simulink model "ob_1_model"  (R2018b)
settings: Solver=VariableStepAuto  StartTime=0.0  StopTime=10.0  RelTol=1e-3
values from neighbouring files (symbols this model uses):
  K = 2    [ob_1.m]    (also in ob_2.m; ob_3.m)
  T_1 = 1    [ob_1.m]    (also in ob_2.m; ob_3.m)
  T_1_a = 0    [ob_1.m]    (also in ob_2.m; ob_3.m)
  T_1_b = T_1/10    (= 0.1)    [ob_1.m]    (also in ob_2.m; ob_3.m)
  T_1_c = T_1/2    (= 0.5)    [ob_1.m]    (also in ob_2.m; ob_3.m)
  T_1_d = T_1*1.05    (= 1.05)    [ob_1.m]    (also in ob_2.m; ob_3.m)
  T_2_a = 0    [ob_1.m]    (also in ob_2.m)
  T_2_b = T_i/100    (= 0.01)    [ob_1.m]    (also in ob_2.m)
  T_2_c = T_i/10    (= 0.1)    [ob_1.m]    (also in ob_2.m)
  T_2_d = T_i*0.99    (= 0.99)    [ob_1.m]    (also in ob_2.m)
  T_2_e = 10*T_i    (= 10)    [ob_1.m]    (also in ob_2.m)
  T_3_a = 0.0001    [ob_1.m]    (also in ob_2.m)
  T_3_b = T_d/100    (= 0.01)    [ob_1.m]    (also in ob_2.m)
  T_3_c = T_d/10    (= 0.1)    [ob_1.m]    (also in ob_2.m)
  T_3_d = T_d*0.99    (= 0.99)    [ob_1.m]    (also in ob_2.m)
  T_d = 1    [ob_1.m]    (also in ob_2.m; ob_3.m = 2.5)
  T_i = 1    [ob_1.m]    (also in ob_2.m)
settings Model: Creator=root  LastModifiedBy=root

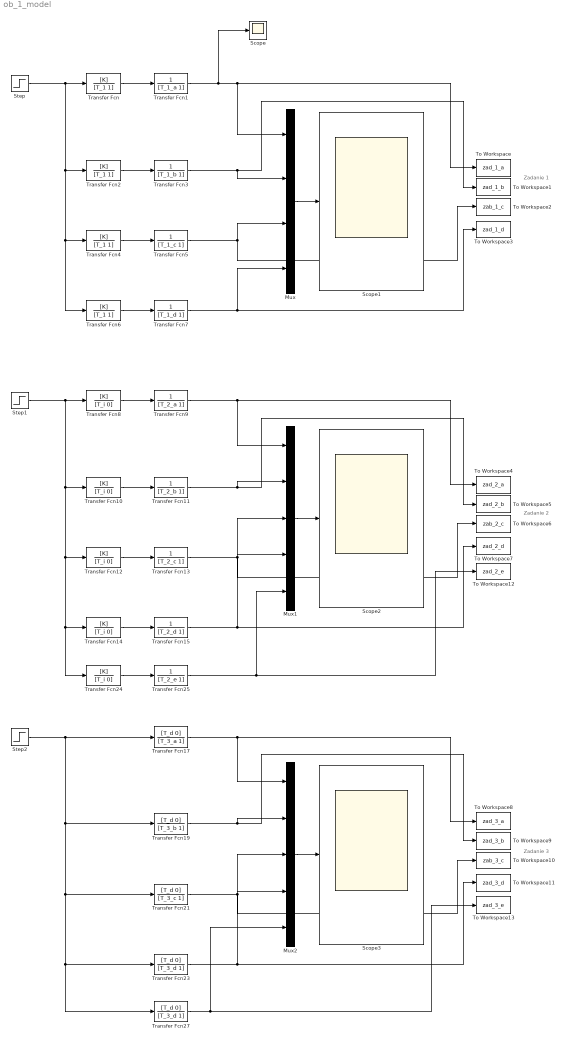
== system ob_1_model ==
  note: Zadanie 3
  note: Zadanie 2
  note: Zadanie 1
  Mux : Mux
  Mux1 : Mux  Inputs=5
  Mux2 : Mux  Inputs=5
  Scope{,1..3} (4 alike) : Scope
  Step : Step  SampleTime=0
  Step1 : Step  SampleTime=0
  Step2 : Step  SampleTime=0
  To Workspace : ToWorkspace  VariableName=zad_1_a  SaveFormat=Timeseries  SampleTime=-1
  To Workspace1 : ToWorkspace  VariableName=zad_1_b  SaveFormat=Timeseries  SampleTime=-1
  To Workspace10 : ToWorkspace  VariableName=zab_3_c  SaveFormat=Timeseries  SampleTime=-1
  To Workspace11 : ToWorkspace  VariableName=zad_3_d  SaveFormat=Timeseries  SampleTime=-1
  To Workspace12 : ToWorkspace  VariableName=zad_2_e  SaveFormat=Timeseries  SampleTime=-1
  To Workspace13 : ToWorkspace  VariableName=zad_3_e  SaveFormat=Timeseries  SampleTime=-1
  To Workspace2 : ToWorkspace  VariableName=zab_1_c  SaveFormat=Timeseries  SampleTime=-1
  To Workspace3 : ToWorkspace  VariableName=zad_1_d  SaveFormat=Timeseries  SampleTime=-1
  To Workspace4 : ToWorkspace  VariableName=zad_2_a  SaveFormat=Timeseries  SampleTime=-1
  To Workspace5 : ToWorkspace  VariableName=zad_2_b  SaveFormat=Timeseries  SampleTime=-1
  To Workspace6 : ToWorkspace  VariableName=zab_2_c  SaveFormat=Timeseries  SampleTime=-1
  To Workspace7 : ToWorkspace  VariableName=zad_2_d  SaveFormat=Timeseries  SampleTime=-1
  To Workspace8 : ToWorkspace  VariableName=zad_3_a  SaveFormat=Timeseries  SampleTime=-1
  To Workspace9 : ToWorkspace  VariableName=zad_3_b  SaveFormat=Timeseries  SampleTime=-1
  Transfer Fcn{,2,4,6} (4 alike) : TransferFcn  Numerator=[K]  Denominator=[T_1 1]
  Transfer Fcn1 : TransferFcn  Denominator=[T_1_a 1]
  Transfer Fcn{8,10,12,14,24} (5 alike) : TransferFcn  Numerator=[K]  Denominator=[T_i 0]
  Transfer Fcn11 : TransferFcn  Denominator=[T_2_b 1]
  Transfer Fcn13 : TransferFcn  Denominator=[T_2_c 1]
  Transfer Fcn15 : TransferFcn  Denominator=[T_2_d 1]
  Transfer Fcn17 : TransferFcn  Numerator=[T_d 0]  Denominator=[T_3_a 1]
  Transfer Fcn19 : TransferFcn  Numerator=[T_d 0]  Denominator=[T_3_b 1]
  Transfer Fcn21 : TransferFcn  Numerator=[T_d 0]  Denominator=[T_3_c 1]
  Transfer Fcn23 : TransferFcn  Numerator=[T_d 0]  Denominator=[T_3_d 1]
  Transfer Fcn25 : TransferFcn  Denominator=[T_2_e 1]
  Transfer Fcn27 : TransferFcn  Numerator=[T_d 0]  Denominator=[T_3_d 1]
  Transfer Fcn3 : TransferFcn  Denominator=[T_1_b 1]
  Transfer Fcn5 : TransferFcn  Denominator=[T_1_c 1]
  Transfer Fcn7 : TransferFcn  Denominator=[T_1_d 1]
  Transfer Fcn9 : TransferFcn  Denominator=[T_2_a 1]
  wires:
  Transfer Fcn/1 -> Transfer Fcn1/1
  Step/1 -> Transfer Fcn6/1, Transfer Fcn4/1, Transfer Fcn2/1, Transfer Fcn/1
  Transfer Fcn2/1 -> Transfer Fcn3/1
  Transfer Fcn4/1 -> Transfer Fcn5/1
  Transfer Fcn6/1 -> Transfer Fcn7/1
  Transfer Fcn1/1 -> Scope/1, To Workspace/1, Mux/1
  Transfer Fcn3/1 -> To Workspace1/1, Mux/2
  Transfer Fcn5/1 -> To Workspace2/1, Mux/3
  Transfer Fcn7/1 -> To Workspace3/1, Mux/4
  Mux/1 -> Scope1/1
  Transfer Fcn12/1 -> Transfer Fcn13/1
  Transfer Fcn10/1 -> Transfer Fcn11/1
  Transfer Fcn13/1 -> To Workspace6/1, Mux1/3
  Transfer Fcn8/1 -> Transfer Fcn9/1
  Transfer Fcn11/1 -> To Workspace5/1, Mux1/2
  Transfer Fcn15/1 -> To Workspace7/1, Mux1/4
  Transfer Fcn9/1 -> To Workspace4/1, Mux1/1
  Mux1/1 -> Scope2/1
  Step1/1 -> Transfer Fcn10/1, Transfer Fcn12/1, Transfer Fcn24/1, Transfer Fcn14/1, Transfer Fcn8/1
  Transfer Fcn14/1 -> Transfer Fcn15/1
  Transfer Fcn21/1 -> To Workspace10/1, Mux2/3
  Step2/1 -> Transfer Fcn17/1, Transfer Fcn19/1, Transfer Fcn21/1, Transfer Fcn23/1, Transfer Fcn27/1
  Transfer Fcn19/1 -> To Workspace9/1, Mux2/2
  Transfer Fcn23/1 -> To Workspace11/1, Mux2/4
  Transfer Fcn17/1 -> To Workspace8/1, Mux2/1
  Mux2/1 -> Scope3/1
  Transfer Fcn25/1 -> To Workspace12/1, Mux1/5
  Transfer Fcn27/1 -> Mux2/5, To Workspace13/1
  Transfer Fcn24/1 -> Transfer Fcn25/1
